simulink model "Arduino_Interface"  (R2024a)
settings: Solver=FixedStepAuto  StartTime=0.0  StopTime=inf  FixedStep=0.01  RelTol=1e-3  EnableMultiTasking=on
libraries: arduinolib x6, arduinosensorlib x1
settings Model: ExtModeTrigDuration=2  Creator=Ingy  LastModifiedBy=legion
settings SolverCC: AutoInsertRateTranBlk=on
settings OptimizationCC: EnhancedBackFolding=on  PassReuseOutputArgsAs=Individual arguments  ZeroExternalMemoryAtStartup=off  ZeroInternalMemoryAtStartup=off  MaxStackSize=64  OptimizeBlockOrder=speed  DifferentSizesBufferReuse=on  OptimizationCustomize=off  EfficientTunableParamExpr=on
settings DebuggingCC: ParameterTunabilityLossMsg=error
settings HardwareCC: ProdBitPerInt=16  ProdBitPerPointer=16  ProdBitPerSizeT=16  ProdBitPerPtrDiffT=16  ProdLargestAtomicFloat=None  ProdWordSize=8  ProdHWDeviceType=Atmel->AVR  UseEmbeddedCoderFeatures=off
settings SFSimCC: MATLABDynamicMemAlloc=off
settings RTWCC: Description=Embedded Coder  SystemTargetFile=ert.tlc  HardwareBoard=Arduino Uno  TemplateMakefile=ert_default_tmf  Toolchain=Arduino AVR  BuildConfiguration=Faster Runs
settings CodeAppCC: ForceParamTrailComments=on  OperatorAnnotations=on  SimulinkDataObjDesc=on  SFDataObjDesc=on  InsertBlockDesc=on
settings ERTTargetCC: SupportContinuousTime=on  SupportNonInlinedSFcns=on  SupportVariableSizeSignals=on  ExtModeTransport=3  ExtModeStaticAlloc=on  ExtModeAutomaticAllocSize=off  ExtModeStaticAllocSize=250  ExtModeMexFile=ext_xcp  ExtModeIntrfLevel=Level2 - Open  ERTSrcFileBannerTemplate=codertarget_code_template.cgt  ERTHdrFileBannerTemplate=codertarget_code_template.cgt  ERTDataSrcFileTemplate=codertarget_code_template.cgt  ERTDataHdrFileTemplate=codertarget_code_template.cgt

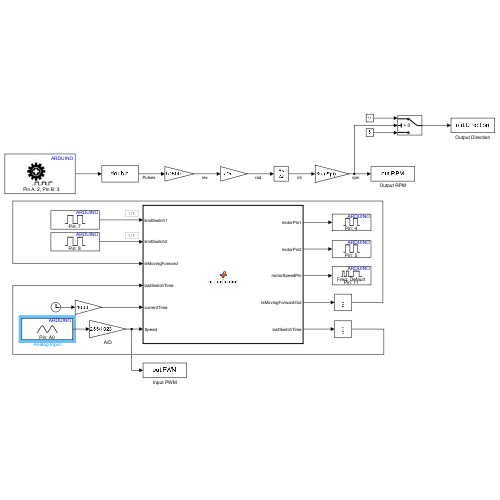
[thumbnail: Simulink's stored preview of the top-level diagram]
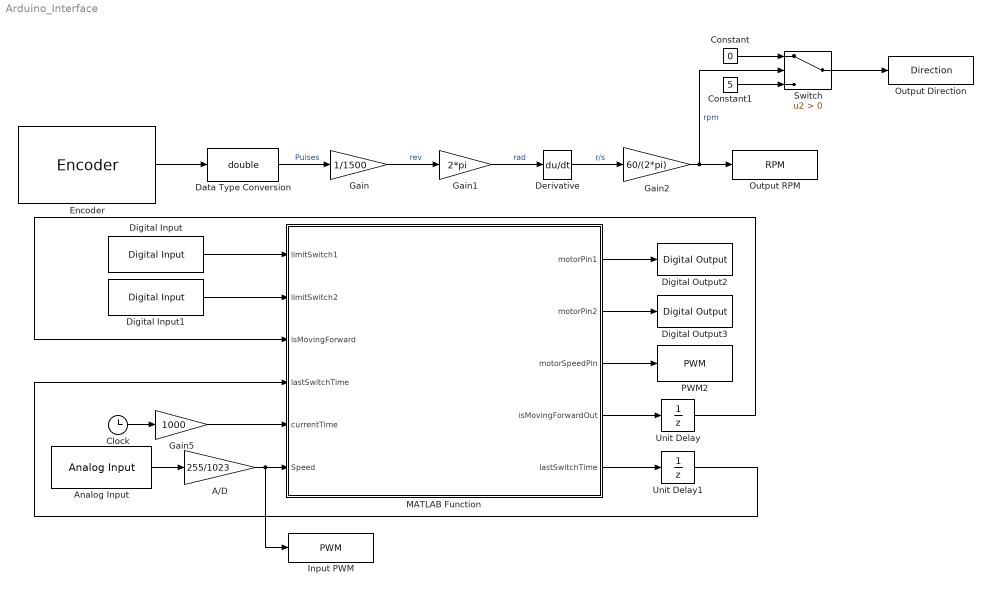
== system Arduino_Interface ==
  A/D : Gain  Gain=255/1023
  Analog Input : arduinolib/Analog Input  pinNumber=0  ReadResultsOnly=off  ConversionTriggerSource=Software  ExternalTriggerType=uint32( 0 )  OutputDataType=uint16  EnableConversionCompleteNotify=off  EnableOuputStatus=off  SampleTime=-1  blockPlatform=arduino
  Clock : Clock
  Constant : Constant  Value=0
  Constant1 : Constant  Value=5
  Data Type Conversion : DataTypeConversion  OutDataTypeStr=double  SaturateOnIntegerOverflow=off  RndMeth=Floor
  Derivative : Derivative
  Digital Input : arduinolib/Digital Input  pinNumber=7  mode=Default  Direction=input  SampleTime=0.1  blockPlatform=arduino
  Digital Input1 : arduinolib/Digital Input  pinNumber=8  mode=Default  Direction=input  SampleTime=0.1  blockPlatform=arduino
  Digital Output2 : arduinolib/Digital Output  pinNumber=4  Direction=output  blockPlatform=arduino
  Digital Output3 : arduinolib/Digital Output  pinNumber=5  Direction=output  blockPlatform=arduino
  Encoder : arduinosensorlib/Encoder  InputA=2  InputB=3  Mode=No reset  SampleTime=-1
  Gain : Gain  Gain=1/1500
  Gain1 : Gain  Gain=2*pi
  Gain2 : Gain  Gain=60/(2*pi)
  Gain5 : Gain  Gain=1000
  Input PWM : ToWorkspace  VariableName=PWM  SaveFormat=Timeseries  SampleTime=-1
  MATLAB Function : MATLAB Function  TreatAsAtomicUnit=on
  Output Direction : ToWorkspace  VariableName=Direction  SaveFormat=Timeseries  SampleTime=-1
      settings: Save2DSignal=2-D array (concatenate along first dimension)
  Output RPM : ToWorkspace  VariableName=RPM  SaveFormat=Timeseries  SampleTime=-1
      settings: Save2DSignal=2-D array (concatenate along first dimension)
  PWM2 : arduinolib/PWM  pinNumber=11  frequencyType=Default  desiredFrequency=490.2  achievableFrequency=490.2
  Switch : Switch  Criteria=u2 > Threshold  SaturateOnIntegerOverflow=off  InputSameDT=off
  Unit Delay : UnitDelay  InitialCondition=1  SampleTime=-1  HasFrameUpgradeWarning=on
  Unit Delay1 : UnitDelay  SampleTime=-1  HasFrameUpgradeWarning=on
  wires:
  Encoder/1 -> Data Type Conversion/1
  Data Type Conversion/1 -> Gain/1  "Pulses"
  Gain/1 -> Gain1/1  "rev"
  Gain1/1 -> Derivative/1  "rad"
  Derivative/1 -> Gain2/1  "r/s"
  Gain2/1 -> Switch/2, Output RPM/1  "rpm"
  Clock/1 -> Gain5/1
  MATLAB Function/5(lastSwitchTime) -> Unit Delay1/1
  Unit Delay1/1 -> MATLAB Function/4("lastSwitchTime ")
  Digital Input/1 -> MATLAB Function/1(limitSwitch1)
  Unit Delay/1 -> MATLAB Function/3(isMovingForward)
  MATLAB Function/3(motorSpeedPin) -> PWM2/1
  MATLAB Function/1(motorPin1) -> Digital Output2/1
  Digital Input1/1 -> MATLAB Function/2(limitSwitch2)
  MATLAB Function/4(isMovingForwardOut) -> Unit Delay/1
  MATLAB Function/2(motorPin2) -> Digital Output3/1
  Gain5/1 -> MATLAB Function/5(currentTime)
  A/D/1 -> Input PWM/1, MATLAB Function/6(Speed)
  Constant/1 -> Switch/1
  Constant1/1 -> Switch/3
  Switch/1 -> Output Direction/1
  Analog Input/1 -> A/D/1

== matlab function Arduino_Interface/MATLAB Function ==
  data: limitSwitch1 input; motorPin1 output; limitSwitch2 input; isMovingForward input; lastSwitchTime input; currentTime input; Speed input; motorPin2 output; motorSpeedPin output; isMovingForwardOut output; lastSwitchTime output
function [motorPin1, motorPin2, motorSpeedPin, isMovingForwardOut, lastSwitchTime] = motorControl(limitSwitch1, limitSwitch2, isMovingForward, lastSwitchTime, currentTime, Speed)
    % Simplified motor control function without delay for immediate start
    
    % Constants and initialization
    motorPin1 = 0;          % Motor Pin 1 (controls forward/reverse direction)
    motorPin2 = 0;          % Motor Pin 2 (controls forward/reverse direction)
    motorSpeedPin = Speed;  % Motor speed (analogWrite equivalent)
    isMovingForwardOut = isMovingForward;  % Initialize direction
    
    % Handle direction logic based on isMovingForward
    if isMovingForward
        % Forward direction logic
        if limitSwitch1 == 1  % If backward limit switch is pressed
            motorPin1 = 0;    % Stop motor
            motorPin2 = 1;    % Reverse direction
            isMovingForwardOut = 0;  % Update direction
        else
            motorPin1 = 1;    % Forward direction
            motorPin2 = 0;    % Forward direction
        end
    else
        % Backward direction logic
        if limitSwitch2 == 1  % If forward limit switch is pressed
            motorPin1 = 1;    % Forward direction
            motorPin2 = 0;    % Forward direction
            isMovingForwardOut = 1;  % Update direction
        else
            motorPin1 = 0;    % Reverse direction
            motorPin2 = 1;    % Reverse direction
        end
    end
    
    % Update lastSwitchTime only when the switch is pressed (for tracking)
    if limitSwitch1 == 1 || limitSwitch2 == 1
        lastSwitchTime = currentTime;
    end
end
